simulink model "DVA_usingcurrent"  (R2020b)
settings: Solver=ode4  StartTime=0.0  StopTime=20  FixedStep=0.001  RelTol=1e-3
model workspace (MAT data in the model file):
  e = 0.05
  k1 = 55666
  k2 = 21012
  m = 0.244
  m1 = 44
  m2 = 5.5
  w = 47.499
libraries: simulink x2
settings Model: Creator=lenovo  LastModifiedBy=lenovo
settings SolverCC: ZeroCrossAlgorithm=Adaptive

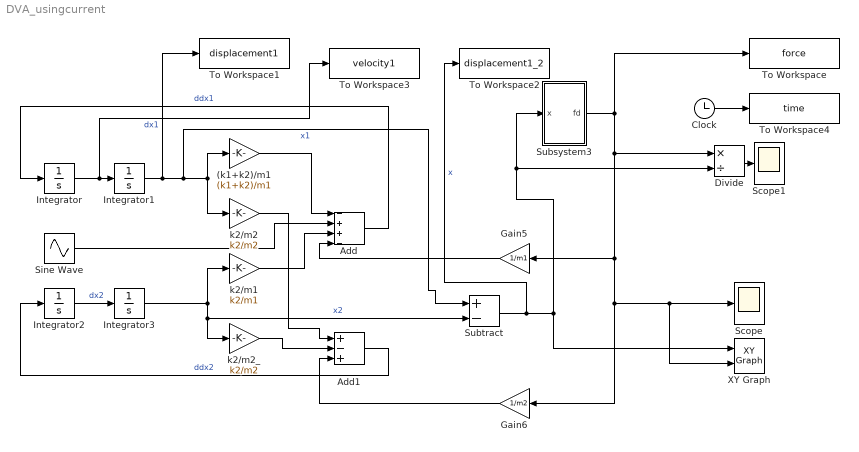
== system DVA_usingcurrent ==
  (k1+k2)/m1 : Gain  Gain=(k1+k2)/m1
  Add : Sum  Inputs=-++-
  Add1 : Sum  Inputs=+-+
  Clock : Clock
  Divide : Product  Inputs=*/
  Gain5 : Gain  Gain=1/m1
  Gain6 : Gain  Gain=1/m2
  Integrator{,1..3} (4 alike) : Integrator
  Scope : Scope
  Scope1 : Scope
  Sine Wave : Sin  Amplitude=(m*e*w^2)/m1  Frequency=w  SampleTime=0
  Subsystem3 : Subsystem
  Subtract : Sum  Inputs=+-
  To Workspace : ToWorkspace  VariableName=force  SampleTime=-1
      settings: Save2DSignal=2-D array (concatenate along first dimension)
  To Workspace1 : ToWorkspace  VariableName=displacement1  SampleTime=-1
      settings: Save2DSignal=2-D array (concatenate along first dimension)
  To Workspace2 : ToWorkspace  VariableName=displacement1_2  SampleTime=-1
      settings: Save2DSignal=2-D array (concatenate along first dimension)
  To Workspace3 : ToWorkspace  VariableName=velocity1  SampleTime=-1
      settings: Save2DSignal=2-D array (concatenate along first dimension)
  To Workspace4 : ToWorkspace  VariableName=time  SampleTime=-1
      settings: Save2DSignal=2-D array (concatenate along first dimension)
  XY Graph : simulink/Sinks/XY Graph  xmin=-5e-5  xmax=0.00012  ymin=-400  ymax=400  st=-1
  k2/m1 : Gain  Gain=k2/m1
  k2/m2 : Gain  Gain=k2/m2
  k2/m2_ : Gain  Gain=k2/m2
  wires:
  Integrator/1 -> To Workspace3/1, Integrator1/1  "dx1"
  Integrator1/1 -> To Workspace1/1, Subtract/1, k2/m2/1, (k1+k2)/m1/1  "x1"
  Integrator2/1 -> Integrator3/1  "dx2"
  Integrator3/1 -> Subtract/2, k2/m2_/1, k2/m1/1  "x2"
  Sine Wave/1 -> Add/2
  k2/m1/1 -> Add/3
  (k1+k2)/m1/1 -> Add/1
  Add/1 -> Integrator/1  "ddx1"
  k2/m2_/1 -> Add1/2
  k2/m2/1 -> Add1/1
  Add1/1 -> Integrator2/1  "ddx2"
  Subtract/1 -> To Workspace2/1, Divide/2, Subsystem3/1(x), XY Graph/1  "x"
  Gain5/1 -> Add/4
  Gain6/1 -> Add1/3
  Subsystem3/1(fd) -> Divide/1, Gain6/1, XY Graph/2, Scope/1, Gain5/1, To Workspace/1
  Divide/1 -> Scope1/1
  Clock/1 -> To Workspace4/1

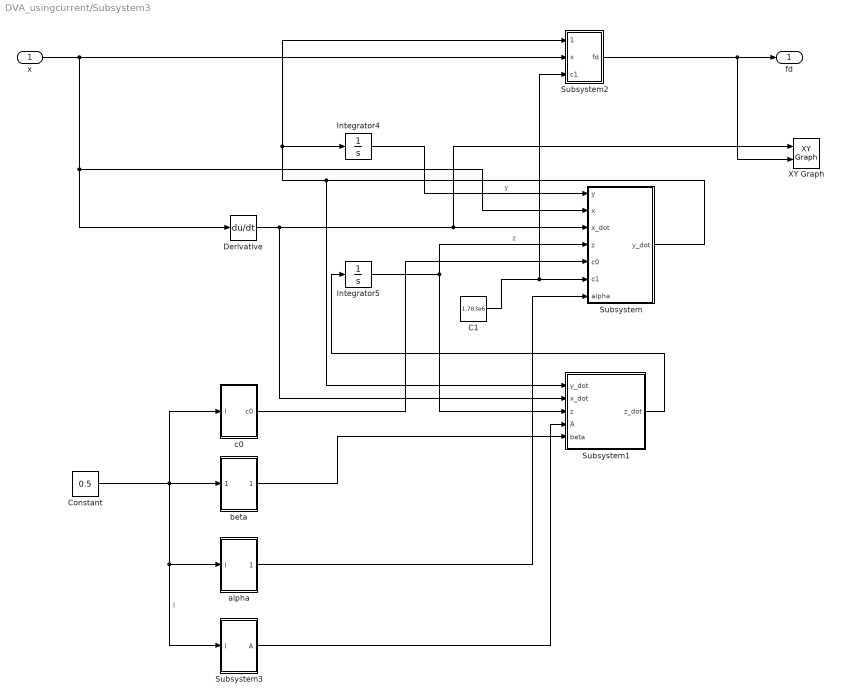
== system DVA_usingcurrent/Subsystem3 ==
  x : Inport
  C1 : Constant  Value=1.783e6
  Constant : Constant  Value=0.5
  Derivative : Derivative
  Integrator4 : Integrator
  Integrator5 : Integrator
  Subsystem : Subsystem
  Subsystem1 : Subsystem
  Subsystem2 : Subsystem
  Subsystem3 : Subsystem
  XY Graph : simulink/Sinks/XY Graph  xmin=-1  xmax=1  ymin=-400  ymax=+400  st=-1
  alpha : Subsystem
  beta : Subsystem
  c0 : Subsystem
  fd : Outport
  wires:
  Subsystem/1(y_dot) -> Subsystem1/1(y_dot), Integrator4/1, Subsystem2/1(y_dot)
  Integrator5/1 -> Subsystem1/3(z), Subsystem/4(z)  "z"
  c0/1(c0) -> Subsystem/5(c0)
  Constant/1 -> c0/1(I), beta/1(In1), Subsystem3/1(I), alpha/1(I)  "I"
  x/1 -> Derivative/1, Subsystem/2(x), Subsystem2/2(x)
  C1/1 -> Subsystem2/3(c1), Subsystem/6(c1)
  Subsystem1/1(z_dot) -> Integrator5/1
  Integrator4/1 -> Subsystem/1(y)  "y"
  Derivative/1 -> Subsystem1/2(x_dot), XY Graph/1, Subsystem/3(x_dot)
  Subsystem2/1(fd) -> XY Graph/2, fd/1
  alpha/1(Out1) -> Subsystem/7(alpha)
  beta/1(Out1) -> Subsystem1/5(beta)
  Subsystem3/1(A) -> Subsystem1/4(A)

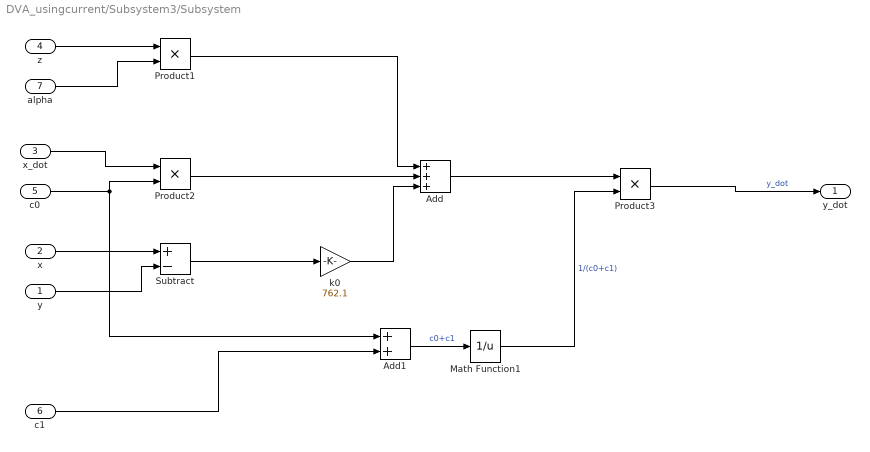
== system DVA_usingcurrent/Subsystem3/Subsystem ==
  y : Inport
  x : Inport  Port=2
  x_dot : Inport  Port=3
  z : Inport  Port=4
  c0 : Inport  Port=5
  c1 : Inport  Port=6
  alpha : Inport  Port=7
  Add : Sum  Inputs=+++
  Add1 : Sum
  Math Function1 : Math  Operator=reciprocal  SaturateOnIntegerOverflow=on
  Product1 : Product
  Product2 : Product
  Product3 : Product
  Subtract : Sum  Inputs=+-
  k0 : Gain  Gain=762.1
  y_dot : Outport
  wires:
  Product1/1 -> Add/1
  Subtract/1 -> k0/1
  Add1/1 -> Math Function1/1  "c0+c1"
  k0/1 -> Add/3
  Math Function1/1 -> Product3/2  "1/(c0+c1)"
  c0/1 -> Add1/1, Product2/2
  z/1 -> Product1/1
  Product3/1 -> y_dot/1  "y_dot"
  Add/1 -> Product3/1
  Product2/1 -> Add/2
  y/1 -> Subtract/2
  x/1 -> Subtract/1
  c1/1 -> Add1/2
  x_dot/1 -> Product2/1
  alpha/1 -> Product1/2

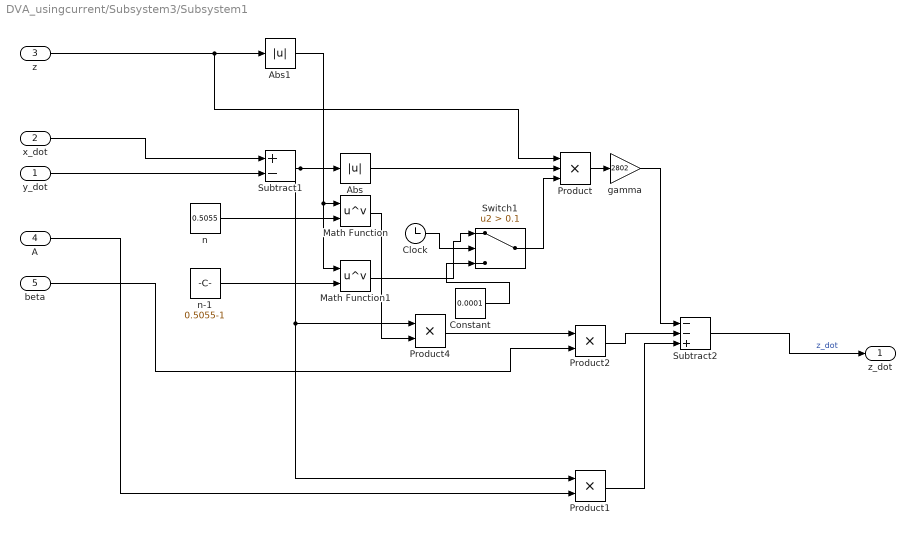
== system DVA_usingcurrent/Subsystem3/Subsystem1 ==
  y_dot : Inport
  x_dot : Inport  Port=2
  z : Inport  Port=3
  A : Inport  Port=4
  beta : Inport  Port=5
  Abs : Abs
  Abs1 : Abs
  Clock : Clock
  Constant : Constant  Value=0.0001
  Math Function : Math  Operator=pow  SaturateOnIntegerOverflow=on
  Math Function1 : Math  Operator=pow  SaturateOnIntegerOverflow=on
  Product : Product  Inputs=3
  Product1 : Product
  Product2 : Product
  Product4 : Product
  Subtract1 : Sum  Inputs=+-
  Subtract2 : Sum  Inputs=--+
  Switch1 : Switch  Criteria=u2 > Threshold  Threshold=0.1
  gamma : Gain  Gain=2802
  n : Constant  Value=0.5055
  n-1 : Constant  Value=0.5055-1
  z_dot : Outport
  wires:
  Abs/1 -> Product/2
  Subtract1/1 -> Product1/1, Product4/1, Abs/1
  n/1 -> Math Function/2
  Abs1/1 -> Math Function1/1, Math Function/1
  gamma/1 -> Subtract2/1
  z/1 -> Abs1/1, Product/1
  Product2/1 -> Subtract2/2
  Product4/1 -> Product2/1
  Math Function/1 -> Product4/2
  Product/1 -> gamma/1
  y_dot/1 -> Subtract1/2
  Subtract2/1 -> z_dot/1  "z_dot"
  x_dot/1 -> Subtract1/1
  Product1/1 -> Subtract2/3
  n-1/1 -> Math Function1/2
  A/1 -> Product1/2
  beta/1 -> Product2/2
  Clock/1 -> Switch1/2
  Switch1/1 -> Product/3
  Constant/1 -> Switch1/3
  Math Function1/1 -> Switch1/1

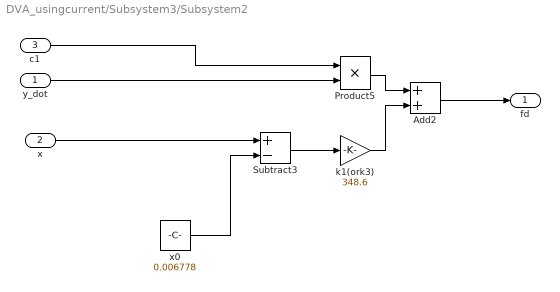
== system DVA_usingcurrent/Subsystem3/Subsystem2 ==
  y_dot : Inport
  x : Inport  Port=2
  c1 : Inport  Port=3
  Add2 : Sum
  Product5 : Product
  Subtract3 : Sum  Inputs=+-
  k1(ork3) : Gain  Gain=348.6
  x0 : Constant  Value=0.006778
  fd : Outport
  wires:
  Subtract3/1 -> k1(ork3)/1
  y_dot/1 -> Product5/2
  Product5/1 -> Add2/1
  k1(ork3)/1 -> Add2/2
  Add2/1 -> fd/1
  x0/1 -> Subtract3/2
  c1/1 -> Product5/1
  x/1 -> Subtract3/1

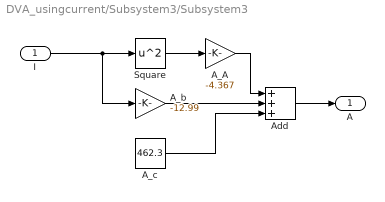
== system DVA_usingcurrent/Subsystem3/Subsystem3 ==
  I : Inport
  A_A : Gain  Gain=-4.367
  A_b : Gain  Gain=-12.99
  A_c : Constant  Value=462.3
  Add : Sum  Inputs=+++
  Square : Math  Operator=square  SaturateOnIntegerOverflow=on
  A : Outport
  wires:
  I/1 -> A_b/1, Square/1
  Square/1 -> A_A/1
  A_b/1 -> Add/2
  A_A/1 -> Add/1
  Add/1 -> A/1
  A_c/1 -> Add/3

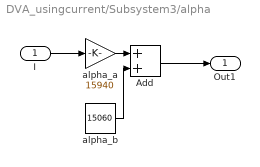
== system DVA_usingcurrent/Subsystem3/alpha ==
  I : Inport
  Add : Sum
  alpha_a : Gain  Gain=15940
  alpha_b : Constant  Value=15060
  Out1 : Outport
  wires:
  I/1 -> alpha_a/1
  alpha_a/1 -> Add/1
  alpha_b/1 -> Add/2
  Add/1 -> Out1/1

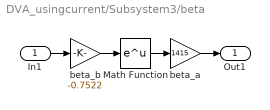
== system DVA_usingcurrent/Subsystem3/beta ==
  In1 : Inport
  Math Function : Math  SaturateOnIntegerOverflow=on
  beta_a : Gain  Gain=1415
  beta_b : Gain  Gain=-0.7522
  Out1 : Outport
  wires:
  In1/1 -> beta_b/1
  beta_b/1 -> Math Function/1
  Math Function/1 -> beta_a/1
  beta_a/1 -> Out1/1

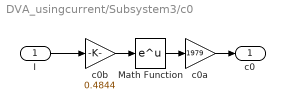
== system DVA_usingcurrent/Subsystem3/c0 ==
  I : Inport
  Math Function : Math  SaturateOnIntegerOverflow=on
  c0a : Gain  Gain=1979
  c0b : Gain  Gain=0.4844
  c0 : Outport
  wires:
  c0b/1 -> Math Function/1
  I/1 -> c0b/1
  c0a/1 -> c0/1
  Math Function/1 -> c0a/1
